simulink model "run_on_QNX_non_inline_sfunc"  (R2017a)
settings: Solver=FixedStepAuto  StartTime=0.0  StopTime=inf  RelTol=1e-3  EnableMultiTasking=on
libraries: simulink x1
settings Model: Creator=darenlee  LastModifiedBy=darenlee
settings SolverCC: PositivePriorityOrder=on
settings OptimizationCC: PassReuseOutputArgsAs=Individual arguments  MaxStackSize=64
settings DebuggingCC: ParameterTunabilityLossMsg=error
settings SFSimCC: MATLABDynamicMemAlloc=off
settings RTWCC: SystemTargetFile=ert.tlc  HardwareBoard=QNX-x86  TLCOptions="-aInlineSetEventsForThisBaseRateFcn=TLC_FALSE -aSuppressMultiTaskScheduler=TLC_FALSE  -aRateBasedStepFcn=0"  TemplateMakefile=ert_default_tmf  Description=Embedded Coder  GenerateReport=on  Toolchain=QNX QCC Toolchain  IncludeHyperlinkInReport=on  LaunchReport=on  GenerateTraceInfo=on  GenerateTraceReport=on  GenerateTraceReportSl=on  GenerateTraceReportSf=on  GenerateTraceReportEml=on
settings CodeAppCC: ForceParamTrailComments=on  IgnoreCustomStorageClasses=off  OperatorAnnotations=on  SimulinkDataObjDesc=on  SFDataObjDesc=on  MATLABFcnDesc=on  InsertBlockDesc=on  MATLABSourceComments=on
settings ERTTargetCC: SupportNonInlinedSFcns=on

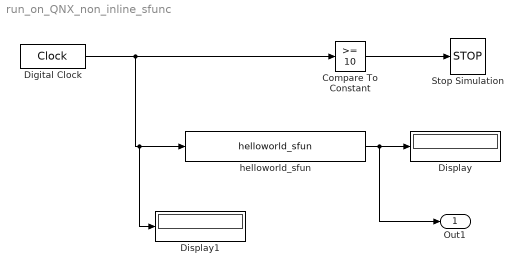
== system run_on_QNX_non_inline_sfunc ==
  Compare To Constant : simulink/Logic and Bit Operations/Compare To Constant  relop=>=  const=10  OutDataTypeStr=boolean
  Digital Clock : DigitalClock
  Display : Display
  Display1 : Display
  Stop Simulation : Stop
  helloworld_sfun : S-Function  FunctionName=helloworld_sfun  SFunctionDeploymentMode=off  EnableBusSupport=off  mask(Legacy Function){SFunctionSpec=double y1 = printValue(double u1), ShowSpec=on}
      mask prompts: ShowSpec "Display function specification"
      mask help:
      | This block allows you to call the legacy functions specified by the following Legacy Code Tool definition:
      | def.SFunctionName = 'helloworld_sfun';
      | def.OutputFcnSpec = 'double y1 = printValue(double u1)';
      | def.StartFcnSpec = 'printValueInit(void)';
      | def.TerminateFcnSpec = 'printValueTerm(void)';
      | def.HeaderFiles = {'hello_world.h'};
      | def.SourceFiles = {'hello_world.c'};
      mask Help: <p>This block was generated automatically by the Legacy Code Tool. For detailed help on this tool, call<a href="matlab:legacy_code('help')"> legacy_code('help')</a>.</p>
      mask Callback ShowSpec:
      | if strcmp(get_param(gcbh, 'ShowSpec'), 'on')
      |   set_param(gcbh, 'MaskDisplay', sprintf('fprintf(''%s'');', get_param(gcbh, 'SFunctionSpec')));
      | else
      |   set_param(gcbh, 'MaskDisplay', sprintf('fprintf(''%s'');', get_param(gcbh, 'FunctionName')));
      | end
      mask Display: fprintf('double y1 = printValue(double u1)');
  Out1 : Outport
  wires:
  Digital Clock/1 -> Compare To Constant/1, Display1/1, helloworld_sfun/1
  helloworld_sfun/1 -> Out1/1, Display/1
  Compare To Constant/1 -> Stop Simulation/1
